simulink model "zad1_rep_gr"  (R2016b)
settings: Solver=VariableStepAuto  StartTime=0.0  StopTime=10.0  RelTol=1e-3
settings Model: Creator=tomasz  LastModifiedBy=tomasz

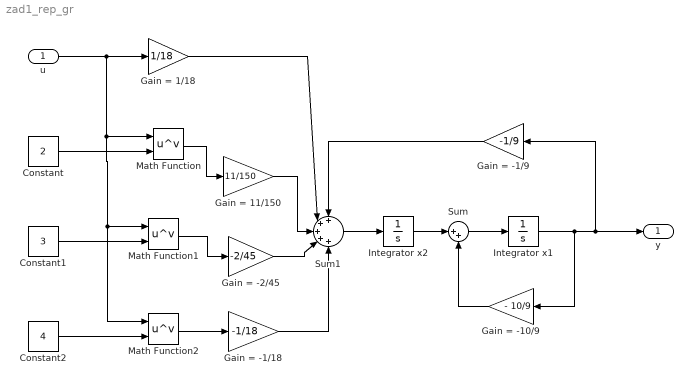
== system zad1_rep_gr ==
  u : Inport
  Constant : Constant  Value=2
  Constant1 : Constant  Value=3
  Constant2 : Constant  Value=4
  Gain = -1/18 : Gain  Gain=-1/18
  Gain = -1/9 : Gain  Gain=-1/9
  Gain = -10/9 : Gain  Gain=- 10/9
  Gain = -2/45 : Gain  Gain=-2/45
  Gain = 1/18 : Gain  Gain=1/18
  Gain = 11/150 : Gain  Gain=11/150
  Integrator x1 : Integrator
  Integrator x2 : Integrator
  Math Function : Math  Operator=pow  SaturateOnIntegerOverflow=on
  Math Function1 : Math  Operator=pow  SaturateOnIntegerOverflow=on
  Math Function2 : Math  Operator=pow  SaturateOnIntegerOverflow=on
  Sum : Sum  Inputs=|++
  Sum1 : Sum  Inputs=+++++
  y : Outport
  wires:
  Sum/1 -> Integrator x1/1
  Integrator x1/1 -> Gain = -1/9/1, y/1, Gain = -10/9/1
  Gain = -10/9/1 -> Sum/2
  Integrator x2/1 -> Sum/1
  Sum1/1 -> Integrator x2/1
  Gain = -1/9/1 -> Sum1/1
  u/1 -> Math Function/1, Math Function2/1, Math Function1/1, Gain = 1/18/1
  Gain = 1/18/1 -> Sum1/2
  Constant1/1 -> Math Function1/2
  Constant2/1 -> Math Function2/2
  Constant/1 -> Math Function/2
  Math Function2/1 -> Gain = -1/18/1
  Math Function1/1 -> Gain = -2/45/1
  Math Function/1 -> Gain = 11/150/1
  Gain = 11/150/1 -> Sum1/3
  Gain = -2/45/1 -> Sum1/4
  Gain = -1/18/1 -> Sum1/5
